simulink model "Linearized_Linear_SS"  (R2019b)
settings: Solver=VariableStepAuto  StartTime=0.0  StopTime=5  RelTol=1e-3
values from neighbouring files (symbols this model uses):
  A = LinearSystem.A    [HOMEWORK..m]
  A_1 = [0 1 0 0 ... (first row only)    [HOMEWORK..m]
  B = LinearSystem.B    [HOMEWORK..m]
  B_1 = [0;-N/(m^2*l^2-M*N);0;(m*l)/(m^2*l^2-M*N)]    [HOMEWORK..m]
  C = [1 0 0 0]    [HOMEWORK..m]
  C_1 = eye(4)    [HOMEWORK..m]
  D = LinearSystem.D    [HOMEWORK..m]
  D_1 = zeros(4,1)    [HOMEWORK..m]
settings Model: Creator=Sina  LastModifiedBy=Harris
settings OptimizationCC: LifeSpan=inf
settings DebuggingCC: SFExecutionAtInitializationDiag=none  ArithmeticOperatorsInVariantConditions=warning
settings SFSimCC: CustomCodeUndefinedFunction=UseInterfaceOnly
settings CodeAppCC: StateflowObjectComments=on

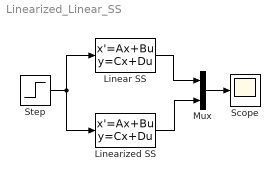
== system Linearized_Linear_SS ==
  Linear SS : StateSpace  A=A_1  B=B_1  C=C_1  D=D_1  InitialCondition=0
  Linearized SS : StateSpace  A=A  B=B  C=C  D=D  InitialCondition=0
  Mux : Mux  Inputs=2
  Scope : Scope
  Step : Step  SampleTime=0
  wires:
  Linearized SS/1 -> Mux/2
  Mux/1 -> Scope/1
  Step/1 -> Linear SS/1, Linearized SS/1
  Linear SS/1 -> Mux/1
